simulink model "calcula_velocidade_manual"  (R2012b)
settings: Solver=FixedStepDiscrete  StartTime=0  StopTime=9.9999  FixedStep=2e-4  MaxStep=1e-4  RelTol=1e-3
libraries: simulink x4, Encoder x1
settings Model: Creator=h3now  LastModifiedBy=h3now
settings DataIOCC: ExternalInput=[time, Hall1, Hall2, Hall3]  LimitDataPoints=off  SaveOutput=off  SaveTime=off

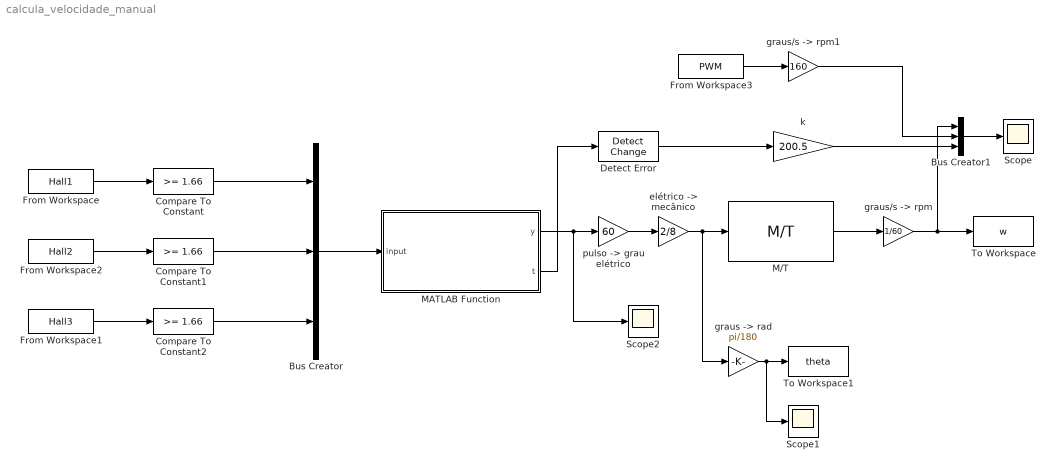
== system calcula_velocidade_manual ==
  Bus Creator : BusCreator  Inputs=3
  Bus Creator1 : BusCreator  Inputs=3
  Compare To Constant : simulink/Logic and Bit Operations/Compare To Constant  relop=>=  const=1.66  OutDataTypeStr=uint8
  Compare To Constant1 : simulink/Logic and Bit Operations/Compare To Constant  relop=>=  const=1.66  OutDataTypeStr=uint8
  Compare To Constant2 : simulink/Logic and Bit Operations/Compare To Constant  relop=>=  const=1.66  OutDataTypeStr=uint8
  Detect Error : simulink/Logic and Bit Operations/Detect Change  vinit=0  InputProcessing=Inherited  OutDataTypeStr=boolean
  From Workspace : FromWorkspace  VariableName=Hall1  SampleTime=0
  From Workspace1 : FromWorkspace  VariableName=Hall3  SampleTime=0
  From Workspace2 : FromWorkspace  VariableName=Hall2  SampleTime=0
  From Workspace3 : FromWorkspace  VariableName=PWM  SampleTime=0
  M/T : Encoder/M//T  Ts=0.02
  MATLAB Function : MATLAB Function  TreatAsAtomicUnit=on
  Scope : Scope
  Scope1 : Scope
  Scope2 : Scope
      settings: SaveName=ScopeData2
  To Workspace : ToWorkspace  VariableName=w  SampleTime=-1
  To Workspace1 : ToWorkspace  VariableName=theta  SampleTime=-1
  "elétrico -> mecânico" : Gain  Gain=2/8
  "graus -> rad" : Gain  Gain=pi/180
  "graus/s -> rpm" : Gain  Gain=1/60
  "graus/s -> rpm1" : Gain  Gain=160
  k : Gain  Gain=200.5  OutDataTypeStr=double
  "pulso -> grau elétrico" : Gain  Gain=60
  wires:
  Bus Creator/1 -> MATLAB Function/1(input)
  From Workspace/1 -> Compare To Constant/1
  From Workspace2/1 -> Compare To Constant1/1
  Compare To Constant/1 -> Bus Creator/1
  Compare To Constant1/1 -> Bus Creator/2
  Compare To Constant2/1 -> Bus Creator/3
  MATLAB Function/1(y) -> Scope2/1, "pulso -> grau elétrico"/1
  "pulso -> grau elétrico"/1 -> "elétrico -> mecânico"/1
  "elétrico -> mecânico"/1 -> "graus -> rad"/1, M/T/1
  M/T/1 -> "graus/s -> rpm"/1
  From Workspace1/1 -> Compare To Constant2/1
  "graus -> rad"/1 -> Scope1/1, To Workspace1/1
  From Workspace3/1 -> "graus/s -> rpm1"/1
  "graus/s -> rpm1"/1 -> Bus Creator1/2
  Bus Creator1/1 -> Scope/1
  MATLAB Function/2(t) -> Detect Error/1
  Detect Error/1 -> k/1
  k/1 -> Bus Creator1/3
  "graus/s -> rpm"/1 -> Bus Creator1/1, To Workspace/1

== matlab function calcula_velocidade_manual/MATLAB Function ==
  data: y output; input input; t output
function [y,t] = state_machine(input)
%#codegen

% A saída t é incrementada de 1 toda vez que ocorrer um erro de transição
% nos Halls

% Initializing persistent variables.
persistent theta;
persistent state;
persistent aux;
if isempty(theta)
    % 'theta' stores the angular position.
    theta = 0; 
    
    aux = 0;
    
    % check starting state and store it in 'state'.
    if isequal(input, [0,0,1]')
        state = 0;
    elseif isequal(input, [1,0,1]')
        state = 1;
    elseif isequal(input, [1,0,0]')
        state = 2;
    elseif isequal(input, [1,1,0]')
        state = 3;
    elseif isequal(input, [0,1,0]')
        state = 4;
    elseif isequal(input, [0,1,1]')
        state = 5;
    else
        state = -1;
    end
        
end

% State machine.
switch state
    case 0
        % keep state.
        if isequal(input,[0,0,1]')
        % go to next state.
        elseif isequal(input,[1,0,1]')
            state = 1;
            theta = theta + 1;
        % go to previous state.
        elseif isequal(input,[0,1,1]')
            state = 5;
            theta = theta - 1;
        % go to error state.
        else
            aux = aux + 1;
        end
        
    case 1
        % keep state.
        if isequal(input,[1,0,1]')
        % go to next state.
        elseif isequal(input,[1,0,0]')
            state = 2;
            theta = theta + 1;
        % go to previous state.
        elseif isequal(input,[0,0,1]')
            state = 0;
            theta = theta - 1;
        % go to error state.
        else
            aux = aux + 1;
        end
        
    case 2
        % keep state.
        if isequal(input,[1,0,0]')
        % go to next state.
        elseif isequal(input,[1,1,0]')
            state = 3;
            theta = theta + 1;
        % go to previous state.
        elseif isequal(input,[1,0,1]')
            state = 1;
            theta = theta - 1;
        % go to error state.
        else
            aux = aux + 1;
        end
        
    case 3
        % keep state.
        if isequal(input,[1,1,0]')
        % go to next state.
        elseif isequal(input,[0,1,0]')
            state = 4;
            theta = theta + 1;
        % go to previous state.
        elseif isequal(input,[1,0,0]')
            state = 2;
            theta = theta - 1;
        % go to error state.
        else
            aux = aux + 1;
        end
        
    case 4
        % keep state.
        if isequal(input,[0,1,0]')
        % go to next state.
        elseif isequal(input,[0,1,1]')
            state = 5;
            theta = theta + 1;
        % go to previous state.
        elseif isequal(input,[1,1,0]')
            state = 3;
            theta = theta - 1;
        % go to error state.
        else
            aux = aux + 1;
        end
        
    case 5
        % keep state.
        if isequal(input,[0,1,1]')
        % go to next state.
        elseif isequal(input,[0,0,1]')
            state = 0;
            theta = theta + 1;
        % go to previous state.
        elseif isequal(input,[0,1,0]')
            state = 4;
            theta = theta - 1;
        % go to error state.
        else
            aux = aux + 1;
        end
        
    case -1
        theta = -32000;
            
end

% Output
y = theta;
t = aux;
